simulink model "moedl1"  (R2020b)
settings: Solver=VariableStepAuto  StartTime=0.0  StopTime=5  RelTol=1e-3
libraries: PoKeysIOInterface x1
settings Model: Creator=64200047  LastModifiedBy=64200047

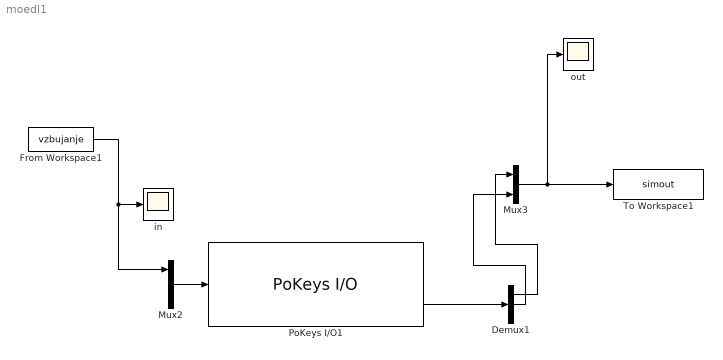
== system moedl1 ==
  Demux1 : Demux  Outputs=3
  From Workspace1 : FromWorkspace  VariableName=vzbujanje
  Mux2 : Mux
  Mux3 : Mux  Inputs=2
  PoKeys I/O1 : PoKeysIOInterface/PoKeys I//O  MaxPowerLimit=100.0  IOTs=0.002  IOSerial=508
      settings: SourceProductName=PoKeys I/O interface
  To Workspace1 : ToWorkspace  VariableName=simout  SaveFormat=Timeseries  SampleTime=-1
  in : Scope
  out : Scope
  wires:
  Mux2/1 -> PoKeys I/O1/1
  PoKeys I/O1/2 -> Demux1/1
  Mux3/1 -> out/1, To Workspace1/1
  Demux1/1 -> Mux3/1
  Demux1/2 -> Mux3/2
  From Workspace1/1 -> Mux2/1, in/1
